simulink model "testemplanner_cs_old"  (R2020a)
settings: Solver=ode5  StartTime=0.0  StopTime=120  FixedStep=1/1000  RelTol=1e-3
PreLoadFcn:
  | mbxruntime.callbacks.PreLoadFcn(bdroot);
PostLoadFcn:
  | mbxruntime.callbacks.PostLoadFcn(bdroot);
InitFcn:
  | mbxruntime.callbacks.InitFcn(bdroot);
StartFcn:
  | mbxruntime.callbacks.StartFcn(bdroot);
StopFcn:
  | mbxruntime.callbacks.StopFcn(bdroot);
model workspace (MAT data in the model file):
  mbox_table : object (value not decoded)
  model_closed = 0
  sim_status = 0
values from neighbouring files (symbols this model uses):
  c_factor = 43.75    [emplanner_init.m]
  cf = -175016    [emplanner_init.m]
  cr = -130634    [emplanner_init.m]
  global_path_x = [0.057304 1.05668625507 2.05480936558 3.05165624935 4.04722112279 5.04150235808 6.03449985569 7.02621407764 8.01664569183 9.00579544113 9.99366409523 10.9802524329 ... (3001 elements, 3001x1)]    [global_path.mat]
  global_path_y = [8.29 8.29 8.29 8.29 8.29 8.29 8.29 8.29 8.29 8.29 8.29 8.29 ... (3001 elements, 3001x1)]    [global_path.mat]
  KD_PID_distance = 0.0    (= 0)    [emplanner_init.m]
  KD_PID_speed = 0    [emplanner_init.m]
  KI_PID_distance = 0.0    (= 0)    [emplanner_init.m]
  KI_PID_speed = 0    [emplanner_init.m]
  KP_PID_distance = 0.5    [emplanner_init.m]
  KP_PID_speed = 1.8    [emplanner_init.m]
  la = 1.265    [emplanner_init.m]
  lb = 2.947-1.265    (= 1.682)    [emplanner_init.m]
  LQR_K1 = k(:,1)'    [emplanner_init.m]
  LQR_K2 = k(:,2)'    [emplanner_init.m]
  LQR_K3 = k(:,3)'    [emplanner_init.m]
  LQR_K4 = k(:,4)'    [emplanner_init.m]
  m = 2020    [emplanner_init.m]
  rack_displacement = [-39.14 , -37.2 , -35.29 , -33.43 , -31.6 , -29.81 , -28.06 , -26.34 , -24.66 ,      -23.01 , -21.38 , -19.79 , -18.23 , -16.69 , -15.18 , -13.7 , -12.23 , -10.8 , -9.38 , -7.98 ,     -6.61 , -5.25 , -3.91 , -2.59 , -1.29 , 0 , 1.27 , 2.54 , 3.78 , 5.02 , 6.24 , 7.46 , 8.66 ,      9.86 , 11.05 , 12.24 , 13.41 , 14.59 , 15.76 , 16.92 , 18.09 , 19.25 , 20.42 , 21.59 , 22.76 ,      23.93 , 25.11 , 26 ...(+26 chars)    [emplanner_init.m]
  right_wheel_ground = [-70 ,-67.2 , -64.4 , -61.6 , -58.8 , -56 , -53.2 , -50.4 , -47.6 , -44.8 , -42 ,      -39.2 , -36.4 , -33.6 , -30.8 , -28 , -25.2 , -22.4 , -19.6 , -16.8 , -14 , -11.2 , -8.4 , -5.6 ,      -2.8 , 0 , 2.8 , 5.6 , 8.4 , 11.2 , 14 , 16.8 , 19.6 , 22.4 , 25.2 , 28 , 30.8 , 33.6 , 36.4 ,      39.2 , 42 , 44.8 , 47.6 , 50.4 , 53.2 , 56 , 58.8 , 61.6 , 64.4 , 67.2 , 70 ]    [emplanner_init.m]
  vx_break_point = zeros(1,5000)    [emplanner_init.m]
undefined symbols (not defined in the file or in its folder): aubr, DiscIntNeverNeededParam, tablebr, vubr
libraries: PreScanSimulinkLibrary x9, Solver_SF x1, simulink_extras x1
(part 3 of 6)

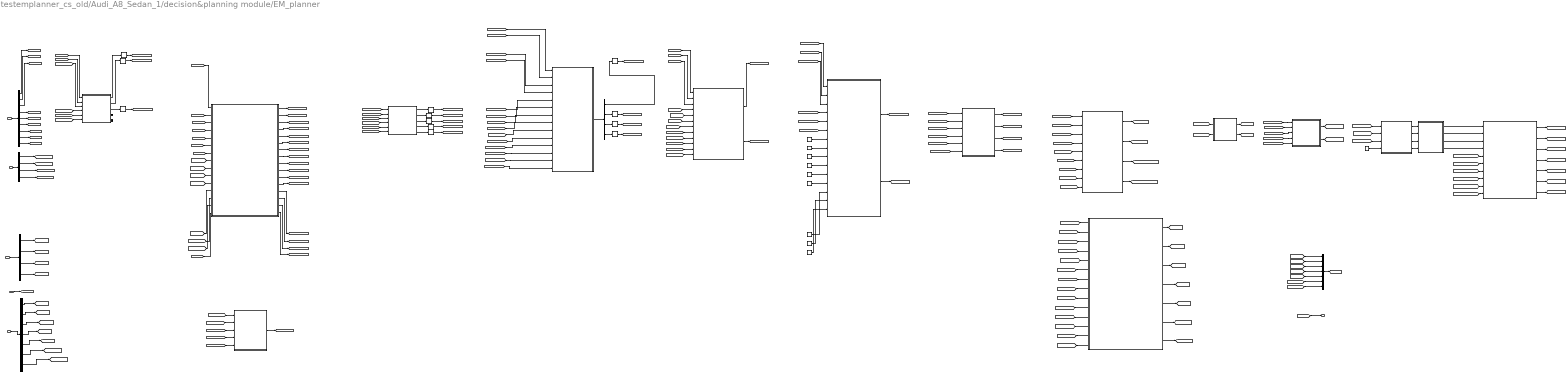
== system testemplanner_cs_old/Audi_A8_Sedan_1/decision&planning module/EM_planner ==
  note: 模块输入整理，输入包括车辆当前位置、航向、速度、加速度信息。参考线信息，车辆在参考线上的投影点信息，感知获取的障碍物信息，当前的时间戳以及上一周期规划出的路径相关信息
  note: 找到规划路径起点，并通过拼接的方式进行平滑
  note: 计算index对应的s，并形成数组，方便进行查阅
  note: 计算规划起点的投影点
  note: 规划起点进行投影
  note: 对障碍物进行筛选和投影
  note: 动态规划主函数
  note: 进行动态规划所求路径的加密，以适应控制的需要
  note: 坐标变换，从Frenet坐标转换为直角坐标，进行控制
  note: 轨迹生成模块
  Location_info : Inport
  referenceline_info : Inport  Port=2
  perceptiong_result : Inport  Port=3
  current_time : Inport  Port=4
  pre_planning_result : Inport  Port=5
  Bus Creator1 : BusCreator  Inputs=7
  Bus Selector : BusSelector  OutputSignals=host_x,host_y,host_heading_xy,host_vx,host_vy,host_yawrate,host_speed,host_ax,host_ay
  Bus Selector1 : BusSelector  OutputSignals=referenceline_x,referenceline_y,path_heading,path_kappa
  Bus Selector2 : BusSelector  OutputSignals=obs_x_set_gcs,obs_y_set_gcs,obs_velocity_set_gcs,obs_heading_set_gcs
  Bus Selector3 : BusSelector  OutputSignals=trajectory_x_final[m],trajectory_y_final[m],trajectory_heading_final[rad],trajectory_kappa_final[1/m],trajectory_velocity_final[m/s],trajectory_accelerate_final[m/s^2],trajectory_time_final[m/s^2]
  Bus Selector4 : BusSelector  OutputSignals=frenet_s_set,frenet_l_set,dl_set,ddl_set
  Cart2Frenet : Subsystem
  Constant9 : Constant  Value=8
  DP node generate : MATLAB Function  TreatAsAtomicUnit=on
  DP path : MATLAB Function  TreatAsAtomicUnit=on
  Frenet2Cart : MATLAB Function  TreatAsAtomicUnit=on
  Index to s : MATLAB Function  TreatAsAtomicUnit=on
  Selector{,1..11} (12 alike) : Selector  InputPortWidth=128  IndexOptions=Index vector (dialog)  Indices=[1]  OutputSizes=1
  Terminator_1 : Terminator
  Terminator_2 : Terminator
  calc path length and map between point and s : MATLAB Function  TreatAsAtomicUnit=on
  calc plan start and stitch trajectory : MATLAB Function  TreatAsAtomicUnit=on
  calc speed planning start condition : MATLAB Function  TreatAsAtomicUnit=on
  col : Constant  Value=4
  general fast algorithm to find projection point info1 : MATLAB Function  TreatAsAtomicUnit=on
  general fast algorithm to find projection point info2 : MATLAB Function  TreatAsAtomicUnit=on
  increase st point count : MATLAB Function  TreatAsAtomicUnit=on
  obs : Subsystem
  path and speed merge : MATLAB Function  TreatAsAtomicUnit=on
  row : Constant  Value=9
  sample_l : Constant
  sample_s : Constant  Value=15
  simple speed qp planning : MATLAB Function  TreatAsAtomicUnit=on
  stitch trajectory : MATLAB Function  TreatAsAtomicUnit=on
  w_collision : Constant  Value=10000
  w_ref : Constant  Value=2000
  w_smooth_dddl : Constant  Value=20
  w_smooth_ddl : Constant  Value=1e8
  w_smooth_dl : Constant  Value=300
  EMplanner_result : Outport
  wires:
  general fast algorithm to find projection point info2/4(proj_heading_set) -> Terminator_1/1
  [trajectory_velocity_final] -> Bus Creator1/5  "trajectory_velocity_final[m/s]"
  [trajectory_x_final] -> Bus Creator1/1  "trajectory_x_final[m]"
  [trajectory_y_final] -> Bus Creator1/2  "trajectory_y_final[m]"
  [referenceline_kappa] -> general fast algorithm to find projection point info2/6(path_kappa)
  general fast algorithm to find projection point info2/2(proj_x_set) -> Selector1/1
  [host_x] -> general fast algorithm to find projection point info2/1(x_set)
  Bus Creator1/1 -> [planning_info]
  [trajectory_accelerate_final] -> Bus Creator1/6  "trajectory_accelerate_final[m/s^2]"
  general fast algorithm to find projection point info2/1(match_point_index_set) -> Selector/1
  [host_y] -> general fast algorithm to find projection point info2/2(y_set)
  [referenceline_x] -> general fast algorithm to find projection point info2/3(path_x)
  general fast algorithm to find projection point info2/5(proj_kappa_set) -> Terminator_2/1
  [referenceline_heading] -> general fast algorithm to find projection point info2/5(path_heading)
  [trajectory_heading_final] -> Bus Creator1/3  "trajectory_heading_final[rad]"
  [referenceline_y] -> general fast algorithm to find projection point info2/4(path_y)
  [trajectory_kappa_final] -> Bus Creator1/4  "trajectory_kappa_final[1/m]"
  general fast algorithm to find projection point info2/3(proj_y_set) -> Selector2/1
  Bus Selector/1 -> [host_x]  "<host_x>"
  Location_info/1 -> Bus Selector/1
  Bus Selector/2 -> [host_y]  "<host_y>"
  referenceline_info/1 -> Bus Selector1/1
  Bus Selector1/4 -> [referenceline_kappa]  "<path_kappa>"
  Bus Selector1/3 -> [referenceline_heading]  "<path_heading>"
  Bus Selector1/2 -> [referenceline_y]  "<referenceline_y>"
  Bus Selector1/1 -> [referenceline_x]  "<referenceline_x>"
  perceptiong_result/1 -> Bus Selector2/1
  Bus Selector2/1 -> [obs_x_set_gcs]  "<obs_x_set_gcs>"
  Bus Selector2/3 -> [obs_velocity_set_gcs]  "<obs_velocity_set_gcs>"
  Bus Selector2/2 -> [obs_y_set_gcs]  "<obs_y_set_gcs>"
  Bus Selector2/4 -> [obs_heading_set_gcs]  "<obs_heading_set_gcs>"
  current_time/1 -> [current_time]
  pre_planning_result/1 -> Bus Selector3/1
  Bus Selector/5 -> [host_vy]  "<host_vy>"
  Bus Selector/6 -> [host_yawrate]  "<host_yawrate>"
  Bus Selector/3 -> [host_heading_xy]  "<host_heading_xy>"
  Bus Selector/4 -> [host_vx]  "<host_vx>"
  Bus Selector/7 -> [host_speed]  "<host_speed>"
  Selector/1 -> [origin_match_point_index]
  Selector1/1 -> [origin_x]
  Selector2/1 -> [origin_y]
  Bus Selector/8 -> [host_ax]  "<host_ax>"
  Bus Selector/9 -> [host_ay]  "<host_ay>"
  [planning_info] -> EMplanner_result/1
  Bus Selector3/6 -> [pre_trajectory_accelerate]  "<trajectory_accelerate_final[m/s^2]>"
  Bus Selector3/1 -> [pre_trajectory_x]  "<trajectory_x_final[m]>"
  Bus Selector3/2 -> [pre_trajectory_y]  "<trajectory_y_final[m]>"
  Bus Selector3/3 -> [pre_trajectory_heading]  "<trajectory_heading_final[rad]>"
  Bus Selector3/4 -> [pre_trajectory_kappa]  "<trajectory_kappa_final[1/m]>"
  Bus Selector3/5 -> [pre_trajectory_velocity]  "<trajectory_velocity_final[m/s]>"
  [trajectory_time_final] -> Bus Creator1/7  "trajectory_time_final[m/s^2]"
  Bus Selector3/7 -> [pre_trajectory_time]  "<trajectory_time_final[m/s^2]>"
  [host_x] -> calc plan start and stitch trajectory/1(host_x)
  [host_y] -> calc plan start and stitch trajectory/2(host_y)
  [host_heading_xy] -> calc plan start and stitch trajectory/3(host_heading_xy)
  [host_vx] -> calc plan start and stitch trajectory/4(host_vx)
  [host_vy] -> calc plan start and stitch trajectory/5(host_vy)
  [host_ax] -> calc plan start and stitch trajectory/6(host_ax)
  [host_ay] -> calc plan start and stitch trajectory/7(host_ay)
  [pre_trajectory_x] -> calc plan start and stitch trajectory/8(pre_trajectory_x)
  [pre_trajectory_heading] -> calc plan start and stitch trajectory/10(pre_trajectory_heading)
  [pre_trajectory_kappa] -> calc plan start and stitch trajectory/11(pre_trajectory_kappa)
  [pre_trajectory_velocity] -> calc plan start and stitch trajectory/12(pre_trajectory_velocity)
  [pre_trajectory_accelerate] -> calc plan start and stitch trajectory/13(pre_trajectory_accelerate)
  [pre_trajectory_time] -> calc plan start and stitch trajectory/14(pre_trajectory_time)
  [pre_trajectory_y] -> calc plan start and stitch trajectory/9(pre_trajectory_y)
  [current_time] -> calc plan start and stitch trajectory/15(current_time)
  calc plan start and stitch trajectory/1(plan_start_x) -> [plan_start_x]
  calc plan start and stitch trajectory/2(plan_start_y) -> [plan_start_y]
  calc plan start and stitch trajectory/3(plan_start_heading) -> [plan_start_heading]
  calc plan start and stitch trajectory/4(plan_start_kappa) -> [plan_start_kappa]
  calc plan start and stitch trajectory/5(plan_start_vx) -> [plan_start_vx]
  calc plan start and stitch trajectory/6(plan_start_vy) -> [plan_start_vy]
  calc plan start and stitch trajectory/7(plan_start_ax) -> [plan_start_ax]
  calc plan start and stitch trajectory/8(plan_start_ay) -> [plan_start_ay]
  calc plan start and stitch trajectory/9(plan_start_time) -> [plan_start_time]
  calc plan start and stitch trajectory/10(stitch_x) -> [stitch_x]
  calc plan start and stitch trajectory/11(stitch_y) -> [stitch_y]
  calc plan start and stitch trajectory/12(stitch_heading) -> [stitch_heading]
  calc plan start and stitch trajectory/13(stitch_kappa) -> [stitch_kappa]
  calc plan start and stitch trajectory/14(stitch_velocity) -> [stitch_velocity]
  calc plan start and stitch trajectory/15(stitch_accelerate) -> [stitch_accelerate]
  calc plan start and stitch trajectory/16(stitch_time) -> [stitch_time]
  [referenceline_x] -> Index to s/1(path_x)
  [referenceline_y] -> Index to s/2(path_y)
  [origin_match_point_index] -> Index to s/5(origin_match_point_index)
  [origin_y] -> Index to s/4(origin_point_y)
  [origin_x] -> Index to s/3(origin_point_x)
  Index to s/1(index2s) -> [index2s]
  Selector5/1 -> [plan_start_proj_y]
  Selector4/1 -> [plan_start_proj_x]
  Selector3/1 -> [plan_start_match_point_index]
  general fast algorithm to find projection point info1/3(proj_y_set) -> Selector5/1
  [referenceline_y] -> general fast algorithm to find projection point info1/4(path_y)
  [referenceline_heading] -> general fast algorithm to find projection point info1/5(path_heading)
  general fast algorithm to find projection point info1/5(proj_kappa_set) -> Selector7/1
  [referenceline_x] -> general fast algorithm to find projection point info1/3(path_x)
  [plan_start_y] -> general fast algorithm to find projection point info1/2(y_set)
  general fast algorithm to find projection point info1/1(match_point_index_set) -> Selector3/1
  [plan_start_x] -> general fast algorithm to find projection point info1/1(x_set)
  general fast algorithm to find projection point info1/2(proj_x_set) -> Selector4/1
  [referenceline_kappa] -> general fast algorithm to find projection point info1/6(path_kappa)
  general fast algorithm to find projection point info1/4(proj_heading_set) -> Selector6/1
  Selector6/1 -> [plan_start_proj_heading]
  Selector7/1 -> [plan_start_proj_kappa]
  [plan_start_x] -> Cart2Frenet/1(plan_start_x)
  [plan_start_y] -> Cart2Frenet/2(plan_start_y)
  [plan_start_vx] -> Cart2Frenet/3(plan_start_vx)
  [plan_start_vy] -> Cart2Frenet/4(plan_start_vy)
  [plan_start_ax] -> Cart2Frenet/5(plan_start_ax)
  [plan_start_ay] -> Cart2Frenet/6(plan_start_ay)
  [referenceline_x] -> Cart2Frenet/7(referenceline_x)
  [referenceline_y] -> Cart2Frenet/8(referenceline_y)
  [index2s] -> Cart2Frenet/9(index2s)
  [plan_start_match_point_index] -> Cart2Frenet/10(plan_start_match_point_index)
  [plan_start_proj_x] -> Cart2Frenet/11(plan_start_proj_x)
  [plan_start_proj_y] -> Cart2Frenet/12(plan_start_proj_y)
  [plan_start_proj_heading] -> Cart2Frenet/13(plan_start_proj_heading)
  [plan_start_proj_kappa] -> Cart2Frenet/14(plan_start_proj_kappa)
  [host_x] -> obs/1(host_x)
  [host_heading_xy] -> obs/3(host_heading_xy)
  [host_y] -> obs/2(host_y)
  [obs_x_set_gcs] -> obs/4(obs_x_set_gcs)
  [obs_y_set_gcs] -> obs/5(obs_y_set_gcs)
  [obs_velocity_set_gcs] -> obs/6(obs_velocity_set_gcs)
  [obs_heading_set_gcs] -> obs/7(obs_heading_set_gcs)
  [referenceline_x] -> obs/8(referenceline_x)
  [referenceline_y] -> obs/9(referenceline_y)
  [referenceline_heading] -> obs/10(referenceline_heading)
  [referenceline_kappa] -> obs/11(referenceline_kappa)
  [index2s] -> obs/12(index2s)
  Cart2Frenet/1(Cart2Frenet_result) -> Bus Selector4/1
  Bus Selector4/1 -> Selector8/1  "<frenet_s_set>"
  Bus Selector4/2 -> Selector9/1  "<frenet_l_set>"
  Bus Selector4/3 -> Selector10/1  "<dl_set>"
  Bus Selector4/4 -> Selector11/1  "<ddl_set>"
  Selector8/1 -> [s_set]
  Selector9/1 -> [l_set]
  Selector10/1 -> [dl_set]
  Selector11/1 -> [ddl_set]
  obs/1(static_obs_s_set) -> [static_obs_s_set]
  obs/2(static_obs_l_set) -> [static_obs_l_set]
  [s_set] -> DP path/1(plan_start_s)
  [l_set] -> DP path/2(plan_start_l)
  [dl_set] -> DP path/3(plan_start_dl)
  [ddl_set] -> DP path/4(plan_start_ddl)
  [static_obs_s_set] -> DP path/5(obs_s_set)
  [static_obs_l_set] -> DP path/6(obs_l_set)
  w_smooth_dl/1 -> DP path/7(w_smooth_dl_cost)
  w_smooth_ddl/1 -> DP path/8(w_collision_cost)
  w_smooth_dddl/1 -> DP path/9(w_ref_cost)
  w_collision/1 -> DP path/11(w_smooth_dddl_cost)
  w_ref/1 -> DP path/10(w_smooth_ddl_cost)
  col/1 -> DP path/12(col)
  row/1 -> DP path/13(row)
  sample_s/1 -> DP path/14(sample_s)
  sample_l/1 -> DP path/15(sample_l)
  DP path/1(dp_path_s_init) -> [dp_path_s_init_set]
  DP path/2(dp_path_l_init) -> [dp_path_l_init_set]
  [dp_path_s_init_set] -> DP node generate/1(dp_path_s_init)
  [dp_path_l_init_set] -> DP node generate/2(dp_path_l_init)
  [s_set] -> DP node generate/3(plan_start_s)
  [l_set] -> DP node generate/4(plan_start_l)
  [dl_set] -> DP node generate/5(plan_start_dl)
  [ddl_set] -> DP node generate/6(plan_start_ddl)
  DP node generate/1(dp_path_s_final) -> [dp_path_s_final]
  DP node generate/4(dp_path_ddl_final) -> [dp_path_ddl_final]
  DP node generate/3(dp_path_dl_final) -> [dp_path_dl_final]
  DP node generate/2(dp_path_l_final) -> [dp_path_l_final]
  [index2s] -> Frenet2Cart/9(index2s)
  [referenceline_kappa] -> Frenet2Cart/8(frenet_kappa)
  [referenceline_heading] -> Frenet2Cart/7(frenet_heading)
  [referenceline_y] -> Frenet2Cart/6(frenet_l)
  [referenceline_x] -> Frenet2Cart/5(frenet_s)
  [dp_path_ddl_final] -> Frenet2Cart/4(ddl_set)
  [dp_path_dl_final] -> Frenet2Cart/3(dl_set)
  [dp_path_l_final] -> Frenet2Cart/2(l_set)
  [dp_path_s_final] -> Frenet2Cart/1(s_set)
  Frenet2Cart/1(x_set) -> [trajectory_x_init]
  Frenet2Cart/2(y_set) -> [trajectory_y_init]
  Frenet2Cart/3(heading_set) -> [trajectory_heading_init]
  Frenet2Cart/4(kappa_set) -> [trajectory_kappa_init]
  [trajectory_x] -> stitch trajectory/1(trajectory_x)
  [trajectory_y] -> stitch trajectory/2(trajectory_y)
  [trajectory_heading] -> stitch trajectory/3(trajectory_heading)
  [trajectory_kappa] -> stitch trajectory/4(trajectory_kappa)
  [trajectory_speed] -> stitch trajectory/5(trajectory_speed)
  [trajectory_accel] -> stitch trajectory/6(trajectory_accel)
  [trajectory_time] -> stitch trajectory/7(trajectory_time)
  [stitch_x] -> stitch trajectory/8(stitch_x)
  [stitch_y] -> stitch trajectory/9(stitch_y)
  [stitch_velocity] -> stitch trajectory/12(stitch_speed)
  [stitch_heading] -> stitch trajectory/10(stitch_heading)
  [stitch_kappa] -> stitch trajectory/11(stitch_kappa)
  [stitch_accelerate] -> stitch trajectory/13(stitch_accel)
  [stitch_time] -> stitch trajectory/14(stitch_time)
  stitch trajectory/1(trajectory_x_final) -> [trajectory_x_final]
  stitch trajectory/2(trajectory_y_final) -> [trajectory_y_final]
  stitch trajectory/3(trajectory_heading_final) -> [trajectory_heading_final]
  stitch trajectory/7(trajectory_time_final) -> [trajectory_time_final]
  stitch trajectory/4(trajectory_kappa_final) -> [trajectory_kappa_final]
  stitch trajectory/5(trajectory_speed_final) -> [trajectory_velocity_final]
  stitch trajectory/6(trajectory_accel_final) -> [trajectory_accelerate_final]
  [plan_start_heading] -> calc speed planning start condition/5(plan_start_heading)
  [plan_start_vx] -> calc speed planning start condition/1(plan_start_vx)
  simple speed qp planning/3(s_dot2_init) -> increase st point count/3(s_dot2_init)
  [trajectory_x_init] -> path and speed merge/7(trajectory_x_init)
  increase st point count/2(s_dot) -> path and speed merge/2(s_dot)
  [plan_start_s_dot2] -> simple speed qp planning/2(plan_start_s_dot2)
  simple speed qp planning/4(relative_time_init) -> increase st point count/4(relative_time_init)
  path and speed merge/7(trajectory_time) -> [trajectory_time]
  [path_s] -> path and speed merge/6(path_s)
  path and speed merge/6(trajectory_accel) -> [trajectory_accel]
  [trajectory_y_init] -> path and speed merge/8(trajectory_y_init)
  [plan_start_ay] -> calc speed planning start condition/4(plan_start_ay)
  increase st point count/4(relative_time) -> path and speed merge/4(relative_time)
  increase st point count/1(s) -> path and speed merge/1(s)
  path and speed merge/1(trajectory_x) -> [trajectory_x]
  [plan_start_ax] -> calc speed planning start condition/3(plan_start_ax)
  calc speed planning start condition/1(plan_start_s_dot) -> [plan_start_s_dot]
  [plan_start_time] -> path and speed merge/5(current_time)
  calc speed planning start condition/2(plan_start_s_dot2) -> [plan_start_s_dot2]
  path and speed merge/2(trajectory_y) -> [trajectory_y]
  simple speed qp planning/2(s_dot_init) -> increase st point count/2(s_dot_init)
  [trajectory_heading_init] -> path and speed merge/9(trajectory_heading_init)
  Constant9/1 -> simple speed qp planning/4(recommend_T)
  path and speed merge/4(trajectory_kappa) -> [trajectory_kappa]
  path and speed merge/3(trajectory_heading) -> [trajectory_heading]
  [plan_start_vy] -> calc speed planning start condition/2(plan_start_vy)
  increase st point count/3(s_dot2) -> path and speed merge/3(s_dot2)
  [trajectory_y_init] -> calc path length and map between point and s/2(trajectory_y)
  simple speed qp planning/1(s_init) -> increase st point count/1(s_init)
  [path_s_end] -> simple speed qp planning/3(s_end)
  [plan_start_s_dot] -> simple speed qp planning/1(plan_start_s_dot)
  path and speed merge/5(trajectory_speed) -> [trajectory_speed]
  calc path length and map between point and s/2(path_s) -> [path_s]
  [trajectory_x_init] -> calc path length and map between point and s/1(trajectory_x)
  [trajectory_kappa_init] -> path and speed merge/10(trajectory_kappa_init)
  calc path length and map between point and s/1(path_s_end) -> [path_s_end]

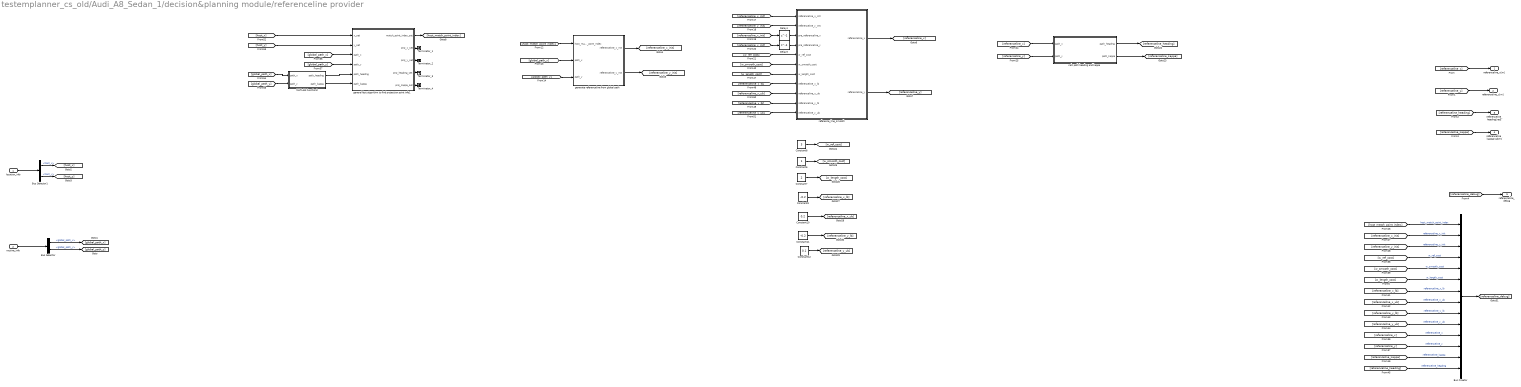
== system testemplanner_cs_old/Audi_A8_Sedan_1/decision&planning module/referenceline provider ==
  location_info : Inport
  routine_info : Inport  Port=2
  Bus Creator : BusCreator  Inputs=14
  Bus Selector : BusSelector  OutputSignals=global_path_x,global_path_y
  Bus Selector1 : BusSelector  OutputSignals=host_x,host_y
  Constant10 : Constant  Value=0.2
  Constant11 : Constant  Value=-0.2
  Constant12 : Constant  Value=0.1
  Constant6 : Constant
  Constant7 : Constant  Value=2
  Constant8 : Constant  Value=3
  Constant9 : Constant  Value=-0.2
  Delay3 : Delay  DelayLength=1
  Delay4 : Delay  DelayLength=1
  MATLAB Function2 : MATLAB Function  TreatAsAtomicUnit=on
  Terminator_{1..4} (4 alike) : Terminator
  calc path heading and kappa : MATLAB Function  TreatAsAtomicUnit=on
  general fast algorithm to find projection point info1 : MATLAB Function  TreatAsAtomicUnit=on
  generate referenceline from global path : MATLAB Function  TreatAsAtomicUnit=on
  reference_line_smooth : MATLAB Function  TreatAsAtomicUnit=on
  referenceline_x[m] : Outport
  referenceline_y[m] : Outport  Port=2
  referenceline_heading[rad] : Outport  Port=3
  referenceline_kappa[rad/m] : Outport  Port=4
  referenceline_debug : Outport  Port=5
  wires:
  [referenceline_x] -> Bus Creator/11  "referenceline_x"
  [referenceline_heading] -> Bus Creator/14  "referenceline_heading"
  Constant12/1 -> [referenceline_y_ub]
  [referenceline_x_ub] -> Bus Creator/8  "referenceline_x_ub"
  Constant10/1 -> [referenceline_x_ub]
  calc path heading and kappa/1(path_heading) -> [referenceline_heading]
  Constant9/1 -> [referenceline_x_lb]
  [w_ref_cost] -> Bus Creator/4  "w_ref_cost"
  [referenceline_y_lb] -> Bus Creator/9  "referenceline_y_lb"
  Constant6/1 -> [w_smooth_cost]
  calc path heading and kappa/2(path_kappa) -> [referenceline_kappa]
  [referenceline_kappa] -> Bus Creator/13  "referenceline_kappa"
  [referenceline_y_init] -> Bus Creator/3  "referenceline_y_init"
  [referenceline_x_lb] -> Bus Creator/7  "referenceline_x_lb"
  Constant7/1 -> [w_length_cost]
  [w_length_cost] -> Bus Creator/6  "w_length_cost"
  [w_smooth_cost] -> Bus Creator/5  "w_smooth_cost"
  Constant8/1 -> [w_ref_cost]
  Constant11/1 -> [referenceline_y_lb]
  [host_match_point_index] -> Bus Creator/1  "host_match_point_index"
  [referenceline_x_init] -> Bus Creator/2  "referenceline_x_init"
  [referenceline_y] -> Bus Creator/12  "referenceline_y"
  [referenceline_y_ub] -> Bus Creator/10  "referenceline_y_ub"
  Bus Creator/1 -> [referenceline_debug]
  routine_info/1 -> Bus Selector/1
  Bus Selector/2 -> [global_path_y]  "<global_path_y>"
  Bus Selector/1 -> [global_path_x]  "<global_path_x>"
  location_info/1 -> Bus Selector1/1
  Bus Selector1/1 -> [host_x]  "<host_x>"
  Bus Selector1/2 -> [host_y]  "<host_y>"
  [referenceline_kappa] -> referenceline_kappa[rad/m]/1
  [referenceline_heading] -> referenceline_heading[rad]/1
  [referenceline_debug] -> referenceline_debug/1
  [referenceline_x] -> referenceline_x[m]/1
  [referenceline_y] -> referenceline_y[m]/1
  [referenceline_x] -> calc path heading and kappa/1(path_x)
  [referenceline_y] -> calc path heading and kappa/2(path_y)
  [host_match_point_index] -> generate referenceline from global path/1(host_match_point_index)
  [global_path_x] -> generate referenceline from global path/2(path_x)
  [global_path_y] -> generate referenceline from global path/3(path_y)
  generate referenceline from global path/2(referenceline_y_init) -> [referenceline_y_init]
  generate referenceline from global path/1(referenceline_x_init) -> [referenceline_x_init]
  [referenceline_x_init] -> reference_line_smooth/1(referenceline_x_init)
  [referenceline_y_init] -> Delay3/1
  [referenceline_x_init] -> Delay4/1
  [referenceline_y_init] -> reference_line_smooth/2(referenceline_y_init)
  Delay3/1 -> reference_line_smooth/4(pre_referenceline_y)
  Delay4/1 -> reference_line_smooth/3(pre_referenceline_x)
  [w_ref_cost] -> reference_line_smooth/5(w_ref_cost)
  [w_smooth_cost] -> reference_line_smooth/6(w_smooth_cost)
  [w_length_cost] -> reference_line_smooth/7(w_length_cost)
  [referenceline_x_lb] -> reference_line_smooth/8(referenceline_x_lb)
  [referenceline_y_lb] -> reference_line_smooth/10(referenceline_y_lb)
  [referenceline_x_ub] -> reference_line_smooth/9(referenceline_x_ub)
  [referenceline_y_ub] -> reference_line_smooth/11(referenceline_y_ub)
  reference_line_smooth/1(referenceline_x) -> [referenceline_x]
  reference_line_smooth/2(referenceline_y) -> [referenceline_y]
  [global_path_y] -> MATLAB Function2/2(path_y)
  [global_path_x] -> MATLAB Function2/1(path_x)
  general fast algorithm to find projection point info1/4(proj_heading_set) -> Terminator_3/1
  general fast algorithm to find projection point info1/2(proj_x_set) -> Terminator_1/1
  general fast algorithm to find projection point info1/3(proj_y_set) -> Terminator_2/1
  [host_x] -> general fast algorithm to find projection point info1/1(x_set)
  MATLAB Function2/1(path_heading) -> general fast algorithm to find projection point info1/5(path_heading)
  MATLAB Function2/2(path_kappa) -> general fast algorithm to find projection point info1/6(path_kappa)
  [global_path_y] -> general fast algorithm to find projection point info1/4(path_y)
  general fast algorithm to find projection point info1/5(proj_kappa_set) -> Terminator_4/1
  [global_path_x] -> general fast algorithm to find projection point info1/3(path_x)
  general fast algorithm to find projection point info1/1(match_point_index_set) -> [host_match_point_index]
  [host_y] -> general fast algorithm to find projection point info1/2(y_set)

== system testemplanner_cs_old/Box_1/Dynamics_Empty/MuxState ==
  note: mode: Dynamics
  note: mode: Positioning
  note: mode: Dynamics
      | VelVEHICLE
      | wrt VEH
  note: AnglesVEHICLE
      | wrtGLOB
  note: For state mode 'Dynamic' positions
      | are not taken into account, as they
      | are computed by integrating velocity.
      | Click annotation for Help.
  x [m] : Inport  SampleTime=TimeStep
  y [m] : Inport  Port=2  SampleTime=TimeStep
  z [m] : Inport  Port=3  SampleTime=TimeStep
  dx [m/s] : Inport  Port=4  SampleTime=TimeStep
  dy [m/s] : Inport  Port=5  SampleTime=TimeStep
  dz [m/s] : Inport  Port=6  SampleTime=TimeStep
  R [rad] : Inport  Port=7  SampleTime=TimeStep
  P [rad] : Inport  Port=8  SampleTime=TimeStep
  Y [rad] : Inport  Port=9  SampleTime=TimeStep
  Constant : Constant  DisableCoverage=on  Value=positioningmode
  Discrete-Time Integrator : DiscreteIntegrator  SampleTime=TimeStep  ICPrevOutput=DiscIntNeverNeededParam  ICPrevScaledInput=DiscIntNeverNeededParam
  Ground : Ground
  Ground1 : Ground
  Mux1 : Mux  Inputs=[3 3]
  Mux2 : Mux  Inputs=3
  Mux3 : Mux  Inputs=3
  Mux4 : Mux  Inputs=3
  Mux5 : Mux  Inputs=[3 3]
  Mux6 : Mux  Inputs=[6 3]
  Switch : Switch  Threshold=0.5
  Transformation_BODY2GLOBAL : PreScanSimulinkLibrary/Simple_Vehicle_Dynamics/Chassis/MuxDynState/Transformation_BODY2GLOBAL  SystemSampleTime=-1  Latency=0  AutoFrameSizeCalculation=off
  mux3 : Mux  Inputs=3
  state : Outport
  wires:
  Constant/1 -> Switch/2
  Mux6/1 -> state/1
  Mux4/1 -> Mux1/1
  Mux5/1 -> Switch/3
  Mux1/1 -> Switch/1
  Switch/1 -> Mux6/1  "PosVeh wrt  GLOB"
  P [rad]/1 -> Mux3/2
  R [rad]/1 -> Mux3/1
  dz [m/s]/1 -> Mux2/3
  dy [m/s]/1 -> Mux2/2
  dx [m/s]/1 -> Mux2/1
  z [m]/1 -> Mux4/3
  y [m]/1 -> Mux4/2
  x [m]/1 -> Mux4/1
  Ground1/1 -> mux3/2  "pitch"
  Y [rad]/1 -> mux3/3, Mux3/3  "yaw"
  Mux3/1 -> Mux6/2
  Transformation_BODY2GLOBAL/1 -> Discrete-Time Integrator/1, Mux5/2  "VelVEH wrt  GLOB"
  mux3/1 -> Transformation_BODY2GLOBAL/2
  Ground/1 -> mux3/1  "roll"
  Mux2/1 -> Mux1/2, Transformation_BODY2GLOBAL/1
  Discrete-Time Integrator/1 -> Mux5/1  "PosVEH wrt  GLOB"

== system testemplanner_cs_old/Box_1/SELF_Demux/compas converter ==
  rotz [rad] : Inport
  cart2compas : Subsystem
  rad2deg : Gain  Gain=180/pi
  heading [deg] : Outport
  wires:
  rad2deg/1 -> cart2compas/1(Angle [deg])
  rotz [rad]/1 -> rad2deg/1
  cart2compas/1(heading [deg]) -> heading [deg]/1

== system testemplanner_cs_old/Audi_A8_Sedan_1/Dynamics_UserSpecified/CarSim2PreScanSTATE/Transformation_SprungMassCarSim2PreScan ==
  In1 : Inport
  Demux : Demux  Outputs=3
  Ini z-position VEHICLE wrt GLOBAL axis system [m] : Constant  Value=z0
  Mux : Mux  Inputs=3
  Sum1 : Sum  Inputs=+-
  Out1 : Outport
  wires:
  Mux/1 -> Out1/1
  Ini z-position VEHICLE wrt GLOBAL axis system [m]/1 -> Sum1/2
  Demux/1 -> Mux/1
  Sum1/1 -> Mux/3
  Demux/3 -> Sum1/1
  Demux/2 -> Mux/2
  In1/1 -> Demux/1

== system testemplanner_cs_old/Audi_A8_Sedan_1/SELF_Demux/compas converter/cart2compas ==
  Angle [deg] : Inport
  Constant : Constant  Value=90
  Constant1 : Constant  Value=360
  Gain : Gain  Gain=1/360
  Gain1 : Gain  Gain=360
  Gain2 : Gain  Gain=-1
  Rounding Function : Rounding
  Sum : Sum  Inputs=|-+
  Sum1 : Sum  Inputs=-+|
  Sum2 : Sum  Inputs=++|
  heading [deg] : Outport
  wires:
  Gain/1 -> Rounding Function/1
  Rounding Function/1 -> Gain1/1
  Gain1/1 -> Sum/1
  Angle [deg]/1 -> Sum1/2
  Sum/1 -> Gain2/1
  Sum1/1 -> Gain/1, Sum/2
  Constant/1 -> Sum1/1
  Gain2/1 -> Sum2/2
  Constant1/1 -> Sum2/1
  Sum2/1 -> heading [deg]/1

== system testemplanner_cs_old/Audi_A8_Sedan_1/Trajectories/Traj2State1/Traj2State2 ==
  traj : Inport
  MuxState : Subsystem
  Traj2MuxState_Ext : Subsystem
  state : Outport
  wires:
  Traj2MuxState_Ext/9(Y [rad]) -> MuxState/9(Y [rad])
  Traj2MuxState_Ext/8(P [rad]) -> MuxState/8(P [rad])
  Traj2MuxState_Ext/7(R [rad]) -> MuxState/7(R [rad])
  Traj2MuxState_Ext/6(dz [m/s]) -> MuxState/6(dz [m/s])
  Traj2MuxState_Ext/5(dy [m/s]) -> MuxState/5(dy [m/s])
  Traj2MuxState_Ext/4(dx [m/s]) -> MuxState/4(dx [m/s])
  Traj2MuxState_Ext/3(z [m]) -> MuxState/3(z [m])
  Traj2MuxState_Ext/2(y [m]) -> MuxState/2(y [m])
  Traj2MuxState_Ext/1(x [m]) -> MuxState/1(x [m])
  MuxState/1(state) -> state/1
  traj/1 -> Traj2MuxState_Ext/1(Traj)

== system testemplanner_cs_old/Audi_A8_Sedan_1/control module1/control main/chassic steering system ==
  LQR_final_angle : Inport
  Constant : Constant  Value=la
  Constant1 : Constant  Value=lb
  Constant17 : Constant  Value=c_factor
  Divide : Product  Inputs=*/
  Gain3 : Gain  Gain=180/pi
  Gain4 : Gain  Gain=360
  MATLAB Function : MATLAB Function  TreatAsAtomicUnit=on
  Saturation : Saturate  UpperLimit=70  LowerLimit=-70
  Saturation1 : Saturate  UpperLimit=1.2217  LowerLimit=-1.2217
  transfer right wheel angle to rack displancement : Lookup_n-D  NumberOfTableDimensions=1  BreakpointsForDimension1=right_wheel_ground  Table=rack_displacement  InternalRulePriority=Speed  RndMeth=Simplest  InputSameDT=on
  lat_steer_sw[deg] : Outport
  wires:
  transfer right wheel angle to rack displancement/1 -> Divide/1
  Constant17/1 -> Divide/2
  Gain4/1 -> lat_steer_sw[deg]/1
  Divide/1 -> Gain4/1
  Saturation/1 -> transfer right wheel angle to rack displancement/1
  Constant/1 -> MATLAB Function/2(la)
  Gain3/1 -> Saturation/1
  Constant1/1 -> MATLAB Function/3(lb)
  LQR_final_angle/1 -> Saturation1/1
  Saturation1/1 -> MATLAB Function/1(u)
  MATLAB Function/1(right_steer) -> Gain3/1

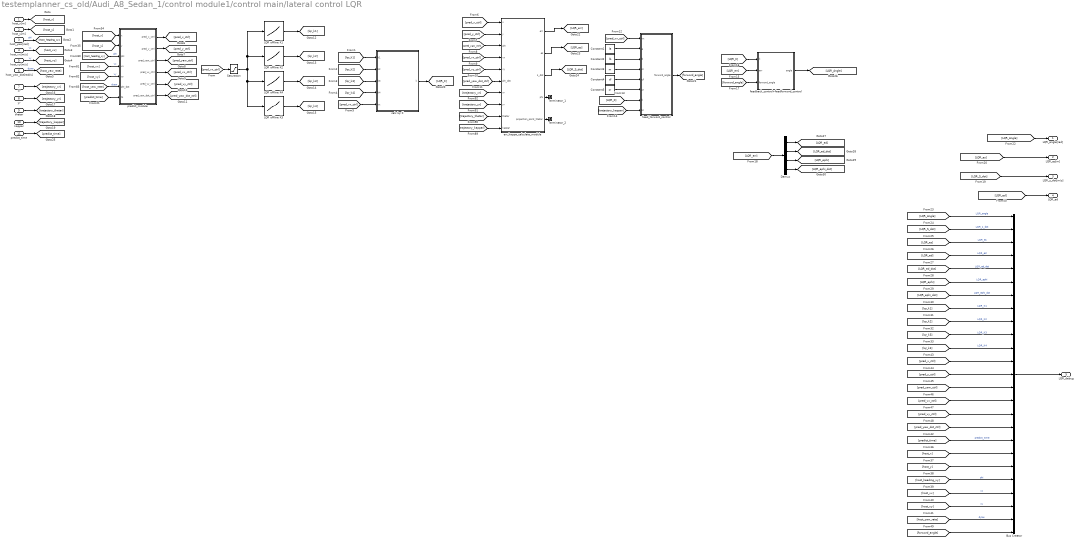
== system testemplanner_cs_old/Audi_A8_Sedan_1/control module1/control main/lateral control LQR ==
  host_x[m] : Inport
  host_y[m] : Inport  Port=2
  host_yaw[rad] : Inport  Port=3
  host_vx[m/s] : Inport  Port=4
  host_vy[m/s] : Inport  Port=5
  host_yaw_dot[rad/s] : Inport  Port=6
  xr : Inport  Port=7
  yr : Inport  Port=8
  thetar : Inport  Port=9
  kappar : Inport  Port=10
  predict_time : Inport  Port=11
  Bus Creator : BusCreator  Inputs=25
  Constant1 : Constant  Value=la
  Constant2 : Constant  Value=lb
  Constant3 : Constant  Value=m
  Constant4 : Constant  Value=cf
  Constant5 : Constant  Value=cr
  Demux : Demux
  LQR offline K1 : Lookup_n-D  NumberOfTableDimensions=1  BreakpointsForDimension1=vx_break_point  Table=LQR_K1  InternalRulePriority=Speed  RndMeth=Simplest  InputSameDT=on
  LQR offline K2 : Lookup_n-D  NumberOfTableDimensions=1  BreakpointsForDimension1=vx_break_point  Table=LQR_K2  InternalRulePriority=Speed  RndMeth=Simplest  InputSameDT=on
  LQR offline K3 : Lookup_n-D  NumberOfTableDimensions=1  BreakpointsForDimension1=vx_break_point  Table=LQR_K3  InternalRulePriority=Speed  RndMeth=Simplest  InputSameDT=on
  LQR offline K4 : Lookup_n-D  NumberOfTableDimensions=1  BreakpointsForDimension1=vx_break_point  Table=LQR_K4  InternalRulePriority=Speed  RndMeth=Simplest  InputSameDT=on
  Saturation : Saturate  UpperLimit=50  LowerLimit=0
  Terminator_1 : Terminator
  Terminator_2 : Terminator
  calc lqr K : MATLAB Function  TreatAsAtomicUnit=on
  err_kappa_calculate_module : MATLAB Function  TreatAsAtomicUnit=on
  feed_forword_control : MATLAB Function  TreatAsAtomicUnit=on
  feedback_control+feedforword_control : MATLAB Function  TreatAsAtomicUnit=on
  predict_module : MATLAB Function  TreatAsAtomicUnit=on
  LQR_angle[rad] : Outport  VectorParamsAs1DForOutWhenUnconnected=off
  LQR_es[m] : Outport  Port=2  VectorParamsAs1DForOutWhenUnconnected=off
  LQR_s_dot[m/s] : Outport  Port=3  VectorParamsAs1DForOutWhenUnconnected=off
  LQR_ed : Outport  Port=4  VectorParamsAs1DForOutWhenUnconnected=off
  LQR_debug : Outport  Port=5  VectorParamsAs1DForOutWhenUnconnected=off
  wires:
  [host_vy] -> predict_module/5(vy)  "vy"
  [host_x] -> predict_module/1(x)
  [host_yaw_rate] -> predict_module/6(phi_dot)  "dyaw"
  [host_vx] -> predict_module/4(vx)  "vx"
  [host_y] -> predict_module/2(y)
  [host_heading_xy] -> predict_module/3(phi)  "phi"
  [predict_time] -> predict_module/7(ts)
  host_x[m]/1 -> [host_x]
  host_y[m]/1 -> [host_y]
  host_yaw[rad]/1 -> [host_heading_xy]  "phi"
  host_vx[m/s]/1 -> [host_vx]  "vx"
  host_vy[m/s]/1 -> [host_vy]  "vy"
  host_yaw_dot[rad/s]/1 -> [host_yaw_rate]  "dyaw"
  predict_module/1(pred_x_ctrl) -> [pred_x_ctrl]
  predict_module/2(pred_y_ctrl) -> [pred_y_ctrl]
  predict_module/3(pred_yaw_ctrl) -> [pred_yaw_ctrl]
  predict_module/4(pred_vx_ctrl) -> [pred_vx_ctrl]
  predict_module/5(pred_vy_ctrl) -> [pred_vy_ctrl]
  predict_module/6(pred_yaw_dot_ctrl) -> [pred_yaw_dot_ctrl]
  [pred_vx_ctrl] -> Saturation/1
  LQR offline K1/1 -> [lqr_k1]
  LQR offline K2/1 -> [lqr_k2]
  LQR offline K4/1 -> [lqr_k3]
  LQR offline K3/1 -> [lqr_k4]
  [pred_vx_ctrl] -> calc lqr K/5(vx)
  [lqr_k4] -> calc lqr K/4(k4)
  [lqr_k3] -> calc lqr K/3(k3)
  [lqr_k2] -> calc lqr K/2(k2)
  [lqr_k1] -> calc lqr K/1(k1)
  [pred_x_ctrl] -> err_kappa_calculate_module/1(x)
  [pred_y_ctrl] -> err_kappa_calculate_module/2(y)
  [pred_yaw_ctrl] -> err_kappa_calculate_module/3("phi ")
  [pred_vx_ctrl] -> err_kappa_calculate_module/4(vx)
  [pred_vy_ctrl] -> err_kappa_calculate_module/5(vy)
  [pred_yaw_dot_ctrl] -> err_kappa_calculate_module/6(phi_dot)
  xr/1 -> [trajectory_xr]
  yr/1 -> [trajectory_yr]
  thetar/1 -> [trajectory_thetar]
  kappar/1 -> [trajectory_kappar]
  [trajectory_xr] -> err_kappa_calculate_module/7(xr)
  [trajectory_yr] -> err_kappa_calculate_module/8(yr)
  [trajectory_kappar] -> err_kappa_calculate_module/10(kappar)
  [trajectory_thetar] -> err_kappa_calculate_module/9(thetar)
  [pred_vx_ctrl] -> feed_forword_control/1(vx)
  Constant1/1 -> feed_forword_control/2(a)
  Constant2/1 -> feed_forword_control/3(b)
  Constant3/1 -> feed_forword_control/4(m)
  Constant4/1 -> feed_forword_control/5(cf)
  Constant5/1 -> feed_forword_control/6(cr)
  calc lqr K/1(k) -> [LQR_K]
  [LQR_K] -> feed_forword_control/7(k)
  [trajectory_kappar] -> feed_forword_control/8(kr)
  feed_forword_control/1(forword_angle) -> [forword_angle]
  err_kappa_calculate_module/1(err) -> [LQR_err]
  [LQR_err] -> feedback_control+feedforword_control/2(err)
  [LQR_K] -> feedback_control+feedforword_control/1(k)
  [forword_angle] -> feedback_control+feedforword_control/3(forword_angle)
  [LQR_err] -> Demux/1
  err_kappa_calculate_module/2(es) -> [LQR_es]
  err_kappa_calculate_module/3(s_dot) -> [LQR_S_dot]
  [LQR_S_dot] -> LQR_s_dot[m/s]/1
  [LQR_es] -> LQR_es[m]/1
  Saturation/1 -> LQR offline K3/1, LQR offline K4/1, LQR offline K2/1, LQR offline K1/1
  predict_time/1 -> [predict_time]
  Bus Creator/1 -> LQR_debug/1
  feedback_control+feedforword_control/1(angle) -> [LQR_Angle]
  [LQR_Angle] -> LQR_angle[rad]/1
  [LQR_Angle] -> Bus Creator/1  "LQR_angle"
  [LQR_S_dot] -> Bus Creator/2  "LQR_s_dot"
  [LQR_es] -> Bus Creator/3  "LQR_es"
  Demux/1 -> [LQR_ed]
  Demux/2 -> [LQR_ed_dot]
  Demux/3 -> [LQR_ephi]
  Demux/4 -> [LQR_ephi_dot]
  [LQR_ed] -> Bus Creator/4  "LQR_ed"
  [LQR_ed_dot] -> Bus Creator/5  "LQR_ed_dot"
  [LQR_ephi] -> Bus Creator/6  "LQR_ephi"
  [LQR_ephi_dot] -> Bus Creator/7  "LQR_ephi_dot"
  [lqr_k1] -> Bus Creator/8  "LQR_K1"
  [lqr_k2] -> Bus Creator/9  "LQR_K2"
  [lqr_k3] -> Bus Creator/10  "LQR_K3"
  [lqr_k4] -> Bus Creator/11  "LQR_K4"
  [pred_x_ctrl] -> Bus Creator/12
  [pred_y_ctrl] -> Bus Creator/13
  [pred_yaw_ctrl] -> Bus Creator/14
  [pred_vx_ctrl] -> Bus Creator/15
  [pred_vy_ctrl] -> Bus Creator/16
  [pred_yaw_dot_ctrl] -> Bus Creator/17
  [predict_time] -> Bus Creator/18  "predict_time"
  [host_x] -> Bus Creator/19
  [host_y] -> Bus Creator/20
  [host_heading_xy] -> Bus Creator/21  "phi"
  [host_vx] -> Bus Creator/22  "vx"
  [host_vy] -> Bus Creator/23  "vy"
  [host_yaw_rate] -> Bus Creator/24  "dyaw"
  [forword_angle] -> Bus Creator/25
  [LQR_ed] -> LQR_ed/1
  err_kappa_calculate_module/4(phi) -> Terminator_1/1
  err_kappa_calculate_module/5(projection_point_thetar) -> Terminator_2/1

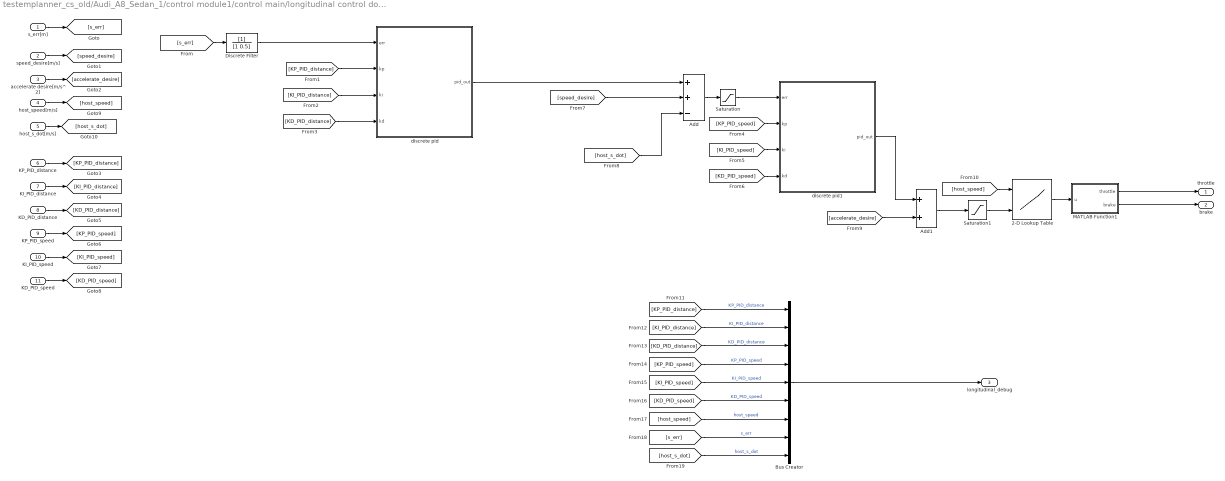
== system testemplanner_cs_old/Audi_A8_Sedan_1/control module1/control main/longitudinal control double PID ==
  s_err[m] : Inport
  speed_desire[m/s] : Inport  Port=2
  accelerate desire[m/s^2] : Inport  Port=3
  host_speed[m/s] : Inport  Port=4
  host_s_dot[m/s] : Inport  Port=5
  KP_PID_distance : Inport  Port=6
  KI_PID_distance : Inport  Port=7
  KD_PID_distance : Inport  Port=8
  KP_PID_speed : Inport  Port=9
  KI_PID_speed : Inport  Port=10
  KD_PID_speed : Inport  Port=11
  2-D Lookup Table : Lookup_n-D  BreakpointsForDimension1=vubr  BreakpointsForDimension2=aubr  Table=tablebr  InternalRulePriority=Speed  RndMeth=Simplest  InputSameDT=on
  Add : Sum  Inputs=++-
  Add1 : Sum
  Bus Creator : BusCreator  Inputs=9
  Discrete Filter : DiscreteFilter
  MATLAB Function1 : MATLAB Function  TreatAsAtomicUnit=on
  Saturation : Saturate  UpperLimit=45  LowerLimit=-45
  Saturation1 : Saturate  UpperLimit=5  LowerLimit=-8
  discrete pid : Subsystem
  discrete pid1 : Subsystem
  throttle : Outport
  brake : Outport  Port=2
  longitudinal_debug : Outport  Port=3
  wires:
  2-D Lookup Table/1 -> MATLAB Function1/1(u)
  s_err[m]/1 -> [s_err]
  speed_desire[m/s]/1 -> [speed_desire]
  accelerate desire[m/s^2]/1 -> [accelerate_desire]
  KP_PID_distance/1 -> [KP_PID_distance]
  KI_PID_distance/1 -> [KI_PID_distance]
  KD_PID_distance/1 -> [KD_PID_distance]
  KP_PID_speed/1 -> [KP_PID_speed]
  KI_PID_speed/1 -> [KI_PID_speed]
  KD_PID_speed/1 -> [KD_PID_speed]
  [s_err] -> Discrete Filter/1
  host_speed[m/s]/1 -> [host_speed]
  [speed_desire] -> Add/2
  Add/1 -> Saturation/1
  Saturation/1 -> discrete pid1/1(err)
  discrete pid1/1(pid_out) -> Add1/1
  [accelerate_desire] -> Add1/2
  Add1/1 -> Saturation1/1
  Saturation1/1 -> 2-D Lookup Table/2
  host_s_dot[m/s]/1 -> [host_s_dot]
  [host_s_dot] -> Add/3
  [host_speed] -> 2-D Lookup Table/1
  MATLAB Function1/1(throttle) -> throttle/1
  MATLAB Function1/2(brake) -> brake/1
  [KP_PID_distance] -> Bus Creator/1  "KP_PID_distance"
  [KI_PID_distance] -> Bus Creator/2  "KI_PID_distance"
  [KD_PID_distance] -> Bus Creator/3  "KD_PID_distance"
  [KP_PID_speed] -> Bus Creator/4  "KP_PID_speed"
  [KI_PID_speed] -> Bus Creator/5  "KI_PID_speed"
  [KD_PID_speed] -> Bus Creator/6  "KD_PID_speed"
  [host_speed] -> Bus Creator/7  "host_speed"
  [s_err] -> Bus Creator/8  "s_err"
  [host_s_dot] -> Bus Creator/9  "host_s_dot"
  Bus Creator/1 -> longitudinal_debug/1
  Discrete Filter/1 -> discrete pid/1(err)
  [KP_PID_distance] -> discrete pid/2(kp)
  [KI_PID_distance] -> discrete pid/3(ki)
  [KD_PID_distance] -> discrete pid/4(kd)
  [KP_PID_speed] -> discrete pid1/2(kp)
  [KI_PID_speed] -> discrete pid1/3(ki)
  [KD_PID_speed] -> discrete pid1/4(kd)
  discrete pid/1(pid_out) -> Add/1

== system testemplanner_cs_old/Audi_A8_Sedan_1/control module1/control main/understeer compensate ==
  LQR_angle : Inport
  lateral err : Inport  Port=2
  Add : Sum  Inputs=+-
  Gain : Gain  Gain=0.01
  Manual Switch : ManualSwitch
  LQR_final_angle : Outport
  wires:
  lateral err/1 -> Gain/1
  Add/1 -> Manual Switch/2
  Manual Switch/1 -> LQR_final_angle/1
  LQR_angle/1 -> Add/1, Manual Switch/1
  Gain/1 -> Add/2

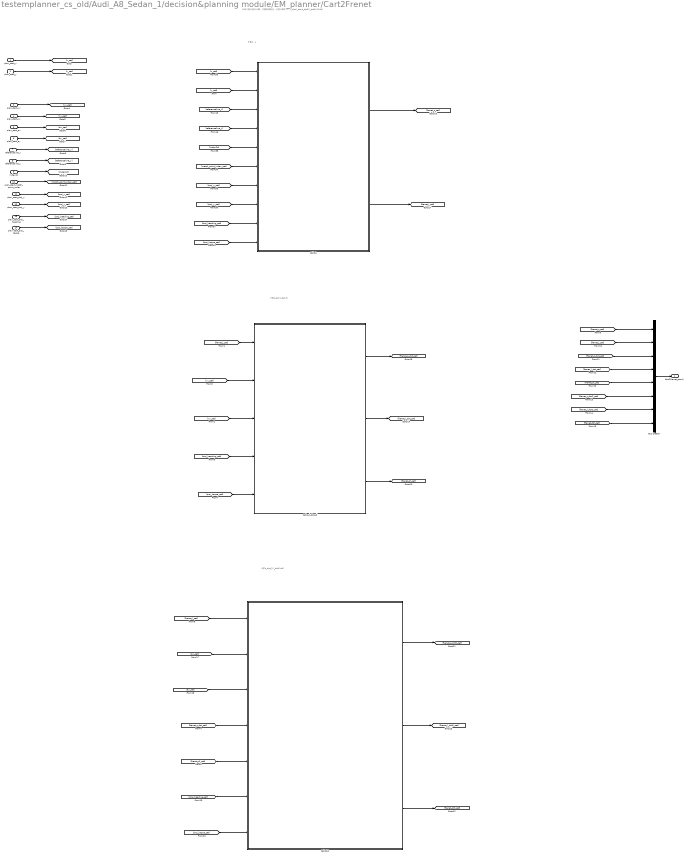
== system testemplanner_cs_old/Audi_A8_Sedan_1/decision&planning module/EM_planner/Cart2Frenet ==
  note: 分成三部分进行计算，方便后续拆分，分别计算S，L，s_dot,l_dot,s_dot2,l_dot2,dl和ddl
  note: 计算S，L
  note: 计算s_dot,l_dot,dl
  note: 计算s_dot_2,l_dot2,ddl
  plan_start_x : Inport
  plan_start_y : Inport  Port=2
  plan_start_vx : Inport  Port=3
  plan_start_vy : Inport  Port=4
  plan_start_ax : Inport  Port=5
  plan_start_ay : Inport  Port=6
  referenceline_x : Inport  Port=7
  referenceline_y : Inport  Port=8
  index2s : Inport  Port=9
  plan_start_match_point_index : Inport  Port=10
  plan_start_proj_x : Inport  Port=11
  plan_start_proj_y : Inport  Port=12
  plan_start_proj_heading : Inport  Port=13
  plan_start_proj_kappa : Inport  Port=14
  Bus Creator : BusCreator  Inputs=8
  CalcSL : MATLAB Function  TreatAsAtomicUnit=on
  CalcSL2 : MATLAB Function  TreatAsAtomicUnit=on
  Calcs_l_dot_dl : MATLAB Function  TreatAsAtomicUnit=on
  Cart2Frenet_result : Outport
  wires:
  CalcSL/1(frenet_s_set) -> [frenet_s_set]
  plan_start_x/1 -> [x_set]
  plan_start_y/1 -> [y_set]
  plan_start_vx/1 -> [vx_set]
  plan_start_vy/1 -> [vy_set]
  plan_start_ax/1 -> [ax_set]
  plan_start_ay/1 -> [ay_set]
  referenceline_x/1 -> [referenceline_x]
  referenceline_y/1 -> [referenceline_y]
  index2s/1 -> [index2s]
  plan_start_match_point_index/1 -> [match_point_index_set]
  plan_start_proj_x/1 -> [proj_x_set]
  plan_start_proj_y/1 -> [proj_y_set]
  plan_start_proj_heading/1 -> [proj_heading_set]
  plan_start_proj_kappa/1 -> [proj_kappa_set]
  [x_set] -> CalcSL/1(x_set)
  [y_set] -> CalcSL/2(y_set)
  [referenceline_x] -> CalcSL/3(referenceline_x)
  [referenceline_y] -> CalcSL/4(referenceline_y)
  [index2s] -> CalcSL/5(index2s)
  [match_point_index_set] -> CalcSL/6(plan_start_match_point_index)
  [proj_x_set] -> CalcSL/7(plan_start_proj_x)
  [proj_y_set] -> CalcSL/8(plan_start_proj_y)
  [proj_heading_set] -> CalcSL/9(plan_start_proj_heading)
  [proj_kappa_set] -> CalcSL/10(plan_start_proj_kappa)
  [proj_kappa_set] -> Calcs_l_dot_dl/5(plan_start_proj_kappa)
  [proj_heading_set] -> Calcs_l_dot_dl/4(plan_start_proj_heading)
  [vx_set] -> Calcs_l_dot_dl/2(vx_set)
  [proj_heading_set] -> CalcSL2/6(plan_start_proj_heading)
  [proj_kappa_set] -> CalcSL2/7(plan_start_proj_kappa)
  CalcSL/2(frenet_l_set) -> [frenet_l_set]
  [frenet_l_set] -> Calcs_l_dot_dl/1(frenet_l_set)
  [vy_set] -> Calcs_l_dot_dl/3(vy_set)
  Calcs_l_dot_dl/1(s_dot_set) -> [frenet_s_dot_set]
  Calcs_l_dot_dl/2(l_dot_set) -> [frenet_l_dot_set]
  Calcs_l_dot_dl/3(dl_set) -> [frenet_dl_set]
  [ax_set] -> CalcSL2/2(ax_set)
  [ay_set] -> CalcSL2/3(ay_set)
  [frenet_dl_set] -> CalcSL2/5(dl_set)
  [frenet_l_set] -> CalcSL2/1(frenet_l_set)
  [frenet_s_dot_set] -> CalcSL2/4(s_dot_set)
  CalcSL2/3(ddl_set) -> [frenet_ddl_set]
  CalcSL2/2(l_dot2_set) -> [frenet_l_dot2_set]
  CalcSL2/1(s_dot2_set) -> [frenet_s_dot2_set]
  [frenet_s_set] -> Bus Creator/1
  [frenet_l_set] -> Bus Creator/2
  [frenet_s_dot_set] -> Bus Creator/3
  [frenet_l_dot_set] -> Bus Creator/4
  [frenet_dl_set] -> Bus Creator/5
  [frenet_s_dot2_set] -> Bus Creator/6
  [frenet_l_dot2_set] -> Bus Creator/7
  [frenet_ddl_set] -> Bus Creator/8
  Bus Creator/1 -> Cart2Frenet_result/1

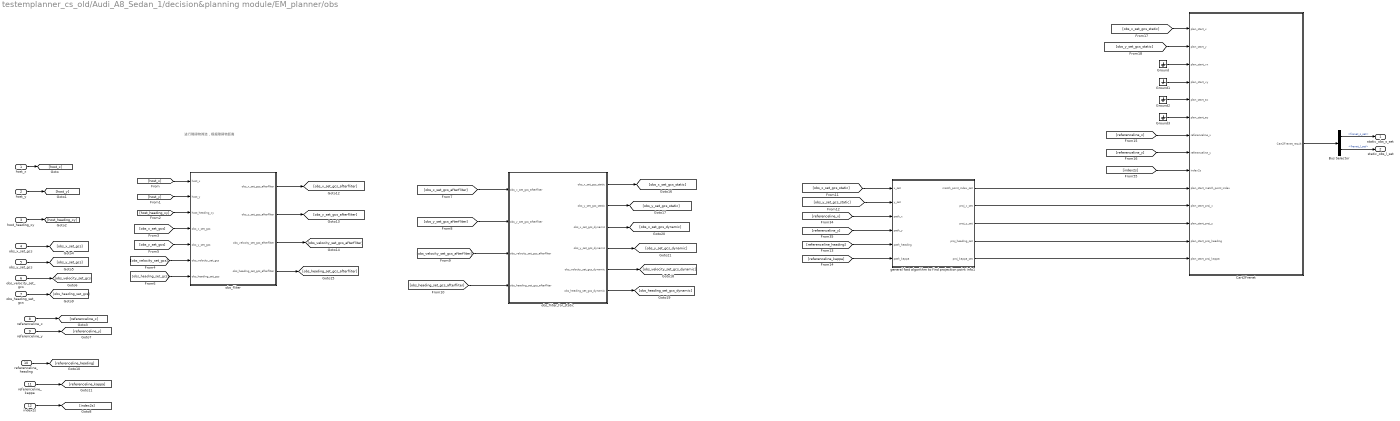
== system testemplanner_cs_old/Audi_A8_Sedan_1/decision&planning module/EM_planner/obs ==
  note: 进行障碍物筛选，根据障碍物距离
  host_x : Inport
  host_y : Inport  Port=2
  host_heading_xy : Inport  Port=3
  obs_x_set_gcs : Inport  Port=4
  obs_y_set_gcs : Inport  Port=5
  obs_velocity_set_gcs : Inport  Port=6
  obs_heading_set_gcs : Inport  Port=7
  referenceline_x : Inport  Port=8
  referenceline_y : Inport  Port=9
  referenceline_heading : Inport  Port=10
  referenceline_kappa : Inport  Port=11
  index2s : Inport  Port=12
  Bus Selector : BusSelector  OutputSignals=frenet_s_set,frenet_l_set
  Cart2Frenet : Subsystem
  Ground{,1..3} (4 alike) : Ground
  general fast algorithm to find projection point info1 : MATLAB Function  TreatAsAtomicUnit=on
  obs_fliter : MATLAB Function  TreatAsAtomicUnit=on
  obs_fliter_for_static : MATLAB Function  TreatAsAtomicUnit=on
  static_obs_s_set : Outport
  static_obs_l_set : Outport  Port=2
  wires:
  [host_x] -> obs_fliter/1(host_x)
  host_x/1 -> [host_x]
  host_y/1 -> [host_y]
  host_heading_xy/1 -> [host_heading_xy]
  obs_x_set_gcs/1 -> [obs_x_set_gcs]
  obs_y_set_gcs/1 -> [obs_y_set_gcs]
  obs_velocity_set_gcs/1 -> [obs_velocity_set_gcs]
  obs_heading_set_gcs/1 -> [obs_heading_set_gcs]
  referenceline_y/1 -> [referenceline_y]
  referenceline_x/1 -> [referenceline_x]
  index2s/1 -> [index2s]
  referenceline_heading/1 -> [referenceline_heading]
  referenceline_kappa/1 -> [referenceline_kappa]
  [obs_heading_set_gcs] -> obs_fliter/7(obs_heading_set_gcs)
  [obs_velocity_set_gcs] -> obs_fliter/6(obs_velocity_set_gcs)
  [obs_y_set_gcs] -> obs_fliter/5(obs_y_set_gcs)
  [obs_x_set_gcs] -> obs_fliter/4(obs_x_set_gcs)
  [host_heading_xy] -> obs_fliter/3(host_heading_xy)
  [host_y] -> obs_fliter/2(host_y)
  obs_fliter/1(obs_x_set_gcs_afterfliter) -> [obs_x_set_gcs_afterfliter]
  obs_fliter/2(obs_y_set_gcs_afterfliter) -> [obs_y_set_gcs_afterfliter]
  obs_fliter/4(obs_heading_set_gcs_afterfliter) -> [obs_heading_set_gcs_afterfliter]
  obs_fliter/3(obs_velocity_set_gcs_afterfliter) -> [obs_velocity_set_gcs_afterfliter]
  [obs_heading_set_gcs_afterfliter] -> obs_fliter_for_static/4(obs_heading_set_gcs_afterfliter)
  [obs_y_set_gcs_afterfliter] -> obs_fliter_for_static/2(obs_y_set_gcs_afterfliter)
  [obs_velocity_set_gcs_afterfliter] -> obs_fliter_for_static/3(obs_velocity_set_gcs_afterfliter)
  [obs_x_set_gcs_afterfliter] -> obs_fliter_for_static/1(obs_x_set_gcs_afterfliter)
  obs_fliter_for_static/1(obs_x_set_gcs_static) -> [obs_x_set_gcs_static]
  obs_fliter_for_static/2(obs_y_set_gcs_static) -> [obs_y_set_gcs_static]
  obs_fliter_for_static/3(obs_x_set_gcs_dynamic) -> [obs_x_set_gcs_dynamic]
  obs_fliter_for_static/4(obs_y_set_gcs_dynamic) -> [obs_y_set_gcs_dynamic]
  obs_fliter_for_static/5(obs_velocity_set_gcs_dynamic) -> [obs_velocity_set_gcs_dynamic]
  obs_fliter_for_static/6(obs_heading_set_gcs_dynamic) -> [obs_heading_set_gcs_dynamic]
  [obs_x_set_gcs_static] -> general fast algorithm to find projection point info1/1(x_set)
  [obs_y_set_gcs_static] -> general fast algorithm to find projection point info1/2(y_set)
  [referenceline_x] -> general fast algorithm to find projection point info1/3(path_x)
  [referenceline_y] -> general fast algorithm to find projection point info1/4(path_y)
  [referenceline_heading] -> general fast algorithm to find projection point info1/5(path_heading)
  [referenceline_kappa] -> general fast algorithm to find projection point info1/6(path_kappa)
  [index2s] -> Cart2Frenet/9(index2s)
  [referenceline_x] -> Cart2Frenet/7(referenceline_x)
  [referenceline_y] -> Cart2Frenet/8(referenceline_y)
  [obs_x_set_gcs_static] -> Cart2Frenet/1(plan_start_x)
  [obs_y_set_gcs_static] -> Cart2Frenet/2(plan_start_y)
  Ground/1 -> Cart2Frenet/3(plan_start_vx)
  Ground3/1 -> Cart2Frenet/6(plan_start_ay)
  Ground2/1 -> Cart2Frenet/5(plan_start_ax)
  Ground1/1 -> Cart2Frenet/4(plan_start_vy)
  general fast algorithm to find projection point info1/1(match_point_index_set) -> Cart2Frenet/10(plan_start_match_point_index)
  general fast algorithm to find projection point info1/2(proj_x_set) -> Cart2Frenet/11(plan_start_proj_x)
  general fast algorithm to find projection point info1/3(proj_y_set) -> Cart2Frenet/12(plan_start_proj_y)
  general fast algorithm to find projection point info1/4(proj_heading_set) -> Cart2Frenet/13(plan_start_proj_heading)
  general fast algorithm to find projection point info1/5(proj_kappa_set) -> Cart2Frenet/14(plan_start_proj_kappa)
  Cart2Frenet/1(Cart2Frenet_result) -> Bus Selector/1
  Bus Selector/1 -> static_obs_s_set/1  "<frenet_s_set>"
  Bus Selector/2 -> static_obs_l_set/1  "<frenet_l_set>"

== system testemplanner_cs_old/Box_1/SELF_Demux/compas converter/cart2compas ==
  Angle [deg] : Inport
  Constant : Constant  Value=90
  Constant1 : Constant  Value=360
  Gain : Gain  Gain=1/360
  Gain1 : Gain  Gain=360
  Gain2 : Gain  Gain=-1
  Rounding Function : Rounding
  Sum : Sum  Inputs=|-+
  Sum1 : Sum  Inputs=-+|
  Sum2 : Sum  Inputs=++|
  heading [deg] : Outport
  wires:
  Gain/1 -> Rounding Function/1
  Rounding Function/1 -> Gain1/1
  Gain1/1 -> Sum/1
  Angle [deg]/1 -> Sum1/2
  Sum/1 -> Gain2/1
  Sum1/1 -> Gain/1, Sum/2
  Constant/1 -> Sum1/1
  Gain2/1 -> Sum2/2
  Constant1/1 -> Sum2/1
  Sum2/1 -> heading [deg]/1

== system testemplanner_cs_old/Audi_A8_Sedan_1/Trajectories/Traj2State1/Traj2State2/MuxState ==
  x [m] : Inport
  y [m] : Inport  Port=2
  z [m] : Inport  Port=3
  dx [m/s] : Inport  Port=4
  dy [m/s] : Inport  Port=5
  dz [m/s] : Inport  Port=6
  R [rad] : Inport  Port=7
  P [rad] : Inport  Port=8
  Y [rad] : Inport  Port=9
  Mux : Mux  Inputs=9
  state : Outport
  wires:
  z [m]/1 -> Mux/3
  y [m]/1 -> Mux/2
  x [m]/1 -> Mux/1
  Y [rad]/1 -> Mux/9
  P [rad]/1 -> Mux/8
  R [rad]/1 -> Mux/7
  dz [m/s]/1 -> Mux/6
  dy [m/s]/1 -> Mux/5
  dx [m/s]/1 -> Mux/4
  Mux/1 -> state/1
